simulink model "benchmark_3"  (R2016a)
settings: Solver=VariableStepAuto  StartTime=0.0  StopTime=time  RelTol=1e-3
values from neighbouring files (symbols this model uses):
  B = 12    [matlab_calc_coupled_v10_valve_area_diff_fric_to_match.m]
  time_step = 0.01    [UAV_LAUNCHER_ASY_working_prot__v10.m]    (also in matlab_calc_actuator.m = 0.1; matlab_calc_tank_side.m = 7.0175)
libraries: fl_lib x21, nesl_utility x7
settings Model: Creator=Engr.Hammad  LastModifiedBy=Engr.Hammad

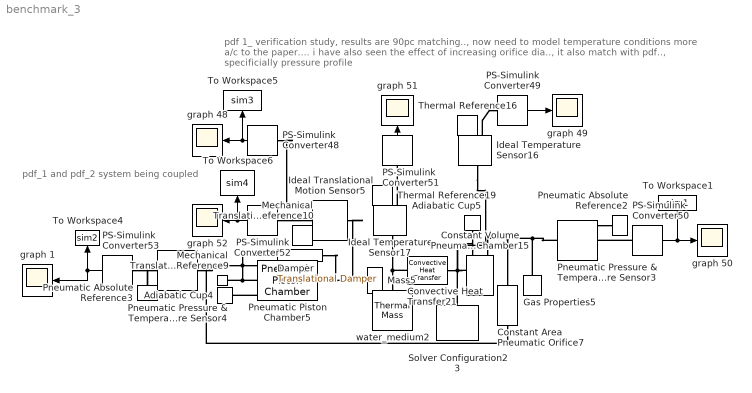
== system benchmark_3 ==
  note: pdf 1_ verification study, results are 90pc   matching.., now need to model temperature conditions more a/c to the paper....
      | i have also seen the effect of increasing orifice dia.., it also match with pdf.., specificially pressure profile
  note: pdf_1 and pdf_2 system being coupled
  Adiabatic Cup4 : fl_lib/Pneumatic/Pneumatic Elements/Adiabatic Cup
  Adiabatic Cup5 : fl_lib/Pneumatic/Pneumatic Elements/Adiabatic Cup
  Constant Area Pneumatic Orifice7 : fl_lib/Pneumatic/Pneumatic Elements/Constant Area Pneumatic Orifice  Cd=1  Area=At m^2  G_specify=off  G_priority=None  G=0 kg/s  Q1_specify=off  Q1_priority=None  Q1=0 J/s  Q2_specify=off  Q2_priority=None  Q2=0 J/s  p1_specify=off  p1_priority=None  p1=1e+5 Pa  p2_specify=off  p2_priority=None  p2=1e+5 Pa  T1_specify=off  T1_priority=None  T1=300 K  T2_specify=off  T2_priority=None  T2=300 K
  Constant Volume Pneumatic Chamber15 : fl_lib/Pneumatic/Pneumatic Elements/Constant Volume Pneumatic Chamber  Volume=V m^3  pressure_specify=on  pressure_priority=High  pressure=P_tank_ini Pa  temperature_specify=on  temperature_priority=High  temperature=T_tank_ini K  gas_flow_specify=off  gas_flow_priority=None  gas_flow=0 kg/s  heat_flow_specify=off  heat_flow_priority=None  heat_flow=0 J/s  heat_exch_flow_specify=off  heat_exch_flow_priority=None  heat_exch_flow=0 J/s
  Convective Heat Transfer21 : fl_lib/Thermal/Thermal Elements/Convective Heat Transfer  area=pi*20*51.5 cm^2  heat_tr_coeff=2321 W/(m^2 * K)  Q_specify=off  Q_priority=None  Q=0 J/s  T_specify=off  T_priority=None  T=0 K
  Damper : fl_lib/Mechanical/Translational Elements/Translational Damper  D=B N/(m/s)  v_specify=off  v_priority=High  v=0 m/s  f_specify=off  f_priority=High  f=0 N
  Gas Properties5 : fl_lib/Pneumatic/Pneumatic Utilities/Gas Properties  c_p=1005 J/kg/K  c_v=717.95 J/kg/K  viscosity=18.21e-6 s*Pa  Pa=101325 Pa  Ta=293.15 K  range_error=2
  Ideal Temperature Sensor16 : fl_lib/Thermal/Thermal Sensors/Ideal Temperature Sensor
  Ideal Temperature Sensor17 : fl_lib/Thermal/Thermal Sensors/Ideal Temperature Sensor
  Ideal Translational Motion Sensor5 : fl_lib/Mechanical/Mechanical Sensors/Ideal Translational Motion Sensor  offset=0 m
  Mass5 : fl_lib/Mechanical/Translational Elements/Mass  mass=M_L kg  v_specify=off  v_priority=High  v=0 m/s  f_specify=off  f_priority=None  f=0 N
  Mechanical Translational Reference10 : fl_lib/Mechanical/Translational Elements/Mechanical Translational Reference
  Mechanical Translational Reference9 : fl_lib/Mechanical/Translational Elements/Mechanical Translational Reference
  PS-Simulink Converter48 : nesl_utility/PS-Simulink Converter  PhysicalDomain=network_engine_domain  SubClassName=ps_output  LeftPortType=input  RightPortType=output  PseudoPeriodic=off  Frequencies=[]  Unit=1  AffineConversion=off
  PS-Simulink Converter49 : nesl_utility/PS-Simulink Converter  PhysicalDomain=network_engine_domain  SubClassName=ps_output  LeftPortType=input  RightPortType=output  PseudoPeriodic=off  Frequencies=[]  Unit=K  AffineConversion=on
  PS-Simulink Converter50 : nesl_utility/PS-Simulink Converter  PhysicalDomain=network_engine_domain  SubClassName=ps_output  LeftPortType=input  RightPortType=output  PseudoPeriodic=off  Frequencies=[]  Unit=1  AffineConversion=on
  PS-Simulink Converter51 : nesl_utility/PS-Simulink Converter  PhysicalDomain=network_engine_domain  SubClassName=ps_output  LeftPortType=input  RightPortType=output  PseudoPeriodic=off  Frequencies=[]  Unit=K  AffineConversion=on
  PS-Simulink Converter52 : nesl_utility/PS-Simulink Converter  PhysicalDomain=network_engine_domain  SubClassName=ps_output  LeftPortType=input  RightPortType=output  PseudoPeriodic=off  Frequencies=[]  Unit=1  AffineConversion=off
  PS-Simulink Converter53 : nesl_utility/PS-Simulink Converter  PhysicalDomain=network_engine_domain  SubClassName=ps_output  LeftPortType=input  RightPortType=output  PseudoPeriodic=off  Frequencies=[]  Unit=1  AffineConversion=off
  Pneumatic Absolute Reference2 : fl_lib/Pneumatic/Pneumatic Elements/Pneumatic Absolute Reference
  Pneumatic Absolute Reference3 : fl_lib/Pneumatic/Pneumatic Elements/Pneumatic Absolute Reference
  Pneumatic Piston Chamber5 : fl_lib/Pneumatic/Pneumatic Elements/Pneumatic Piston Chamber  Area=pis_area m^2  x0=0 m  V0=V0 m^3  or=1  pressure_specify=on  pressure_priority=High  pressure=P0 Pa  temperature_specify=on  temperature_priority=High  temperature=Tc K  gas_flow_specify=off  gas_flow_priority=None  gas_flow=0 kg/s  heat_flow_specify=off  heat_flow_priority=None  heat_flow=0 J/s  heat_exch_flow_specify=off  heat_exch_flow_priority=None  heat_exch_flow=0 J/s  velocity_specify=off  velocity_priority=None  velocity=0 m/s  force_specify=off  force_priority=None  force=0 N
  Pneumatic Pressure & Temperature Sensor3 : fl_lib/Pneumatic/Pneumatic Sensors/Pneumatic Pressure & Temperature Sensor
  Pneumatic Pressure & Temperature Sensor4 : fl_lib/Pneumatic/Pneumatic Sensors/Pneumatic Pressure & Temperature Sensor
  Solver Configuration23 : nesl_utility/Solver Configuration  PhysicalDomain=network_engine_domain  SubClassName=solver  LeftPortType=input  RightPortType=generic  Accelerate=off  Tones=[]  Harmonics=[]  SimulateNoise=off  Profile=off  UseLocalSampling=off  EnableSwitchedLinearOptims=on  FrequencyDomain=off  UseCCode=off  RelTol=0.001  AbsTol=1e-06  MinStep=1e-09  ToWorkspace=off  RevertToSquareIcSolve=off  NumHomotopyIterations=100  PhasorMode=off  PhasorModeNumHarmonics=1  OverrideAbsTol=off  DoDC=off  ResidualTolerance=1e-09  UseLocalSolver=off  LocalSolverChoice=NE_BACKWARD_EULER_ADVANCER  LocalSolverSampleTime=0.001  DoFixedCost=off  MaxNonlinIter=3  MaxModeIter=2  LinearAlgebra=Sparse  DelaysMemoryBudget=1024  AutomaticFiltering=on  FilteringTimeConstant=0.001
  Thermal Reference16 : fl_lib/Thermal/Thermal Elements/Thermal Reference
  Thermal Reference19 : fl_lib/Thermal/Thermal Elements/Thermal Reference
  To Workspace1 : ToWorkspace  VariableName=sim1  SaveFormat=Structure With Time  SampleTime=time_step
  To Workspace4 : ToWorkspace  VariableName=sim2  SaveFormat=Structure With Time  SampleTime=time_step
  To Workspace5 : ToWorkspace  VariableName=sim3  SaveFormat=Structure With Time  SampleTime=time_step
  To Workspace6 : ToWorkspace  VariableName=sim4  SaveFormat=Structure With Time  SampleTime=time_step
  graph {1,48..52} (6 alike) : Scope
  water_medium2 : fl_lib/Thermal/Thermal Elements/Thermal Mass  mass=34334343432 kg  sp_heat=1000 J/kg/K  T_specify=on  T_priority=High  T=20 degC  Q_specify=off  Q_priority=None  Q=0 J/s
  wires:
  PS-Simulink Converter49/1 -> graph 49/1
  PS-Simulink Converter50/1 -> To Workspace1/1, graph 50/1
  PS-Simulink Converter51/1 -> graph 51/1
  PS-Simulink Converter48/1 -> graph 48/1, To Workspace5/1
  PS-Simulink Converter52/1 -> To Workspace6/1, graph 52/1
  PS-Simulink Converter53/1 -> To Workspace4/1, graph 1/1
  connections:
  Pneumatic Pressure & Temperature Sensor3/LConn1 -- Gas Properties5/RConn1 -- Constant Area Pneumatic Orifice7/LConn1 -- Constant Volume Pneumatic Chamber15/LConn1
  Convective Heat Transfer21/LConn1 -- Solver Configuration23/RConn1 -- Ideal Temperature Sensor16/LConn1 -- Adiabatic Cup5/LConn1 -- Constant Volume Pneumatic Chamber15/LConn2
  Convective Heat Transfer21/RConn1 -- water_medium2/LConn1 -- Ideal Temperature Sensor17/LConn1
  Mass5/LConn1 -- Ideal Translational Motion Sensor5/LConn1 -- Damper/LConn1 -- Pneumatic Piston Chamber5/RConn1
  Pneumatic Piston Chamber5/LConn1 -- Pneumatic Pressure & Temperature Sensor4/LConn1 -- Constant Area Pneumatic Orifice7/RConn1
  Pneumatic Pressure & Temperature Sensor3/RConn1 -- Pneumatic Absolute Reference2/LConn1
  PS-Simulink Converter53/LConn1 -- Pneumatic Pressure & Temperature Sensor4/RConn2
  Pneumatic Absolute Reference3/LConn1 -- Pneumatic Pressure & Temperature Sensor4/RConn1
  Thermal Reference19/LConn1 -- Ideal Temperature Sensor17/RConn1
  Ideal Translational Motion Sensor5/RConn1 -- Mechanical Translational Reference10/LConn1
  Ideal Temperature Sensor16/RConn2 -- PS-Simulink Converter49/LConn1
  Pneumatic Piston Chamber5/LConn3 -- Adiabatic Cup4/LConn1
  Thermal Reference16/LConn1 -- Ideal Temperature Sensor16/RConn1
  PS-Simulink Converter48/LConn1 -- Ideal Translational Motion Sensor5/RConn3
  Ideal Temperature Sensor17/RConn2 -- PS-Simulink Converter51/LConn1
  Pneumatic Piston Chamber5/LConn2 -- Damper/RConn1 -- Mechanical Translational Reference9/LConn1
  PS-Simulink Converter50/LConn1 -- Pneumatic Pressure & Temperature Sensor3/RConn2
  PS-Simulink Converter52/LConn1 -- Ideal Translational Motion Sensor5/RConn2
